simulink library "CarMaker4SL"  (R2021a)
settings: Solver=ode45  StartTime=0.0  StopTime=10.0  RelTol=1e-3
libraries: simulink x1
(part 1 of 3)
settings Model: ModifiedByFormat=IPG  ExtModeAutoUpdateStatusClock=off  Creator=IPG  LastModifiedBy=IPG
settings SolverCC: AlgebraicLoopSolver=TrustRegion
settings DataIOCC: LimitDataPoints=on  SaveFormat=Array  SignalLoggingSaveFormat=ModelDataLogs  ReturnWorkspaceOutputs=off
settings OptimizationCC: BlockReduction=off  BooleanDataType=off  ExpressionDepthLimit=2147483647  LifeSpan=inf
settings DebuggingCC: SaveWithParameterizedLinksMsg=none  UnderspecifiedInitializationDetection=Classic  MergeDetectMultiDrivingBlocksExec=none  SignalResolutionControl=TryResolveAllWithWarning  FcnCallInpInsideContextMsg=warning  StateNameClashWarn=warning  SFUnexpectedBacktrackingDiag=warning  SFNoUnconditionalDefaultTransitionDiag=warning  SFMachineParentedDataDiag=warning  ArithmeticOperatorsInVariantConditions=warning
settings HardwareCC: ProdBitPerPointer=32  ProdBitPerSizeT=32  ProdBitPerPtrDiffT=32  ProdLargestAtomicFloat=None  ProdIntDivRoundTo=Undefined  ProdEndianess=Unspecified  ProdWordSize=32  ProdHWDeviceType=32-bit Generic  TargetUnknown=on
settings ModelReferenceCC: PropagateSignalLabelsOutOfModel=off
settings SFSimCC: SimUseLocalCustomCode=off  CustomCodeUndefinedFunction=UseInterfaceOnly
settings RTWCC: RTWUseLocalCustomCode=off
settings CodeAppCC: StateflowObjectComments=on
settings GRTTargetCC: TargetLangStandard=C89/C90 (ANSI)  CombineOutputUpdateFcns=off  GRTInterface=on
settings ConfigComp: CovMetricSettings=dw  CovSaveCumulativeToWorkspaceVar=on  CovSaveSingleToWorkspaceVar=on  CovExternalEMLEnable=off

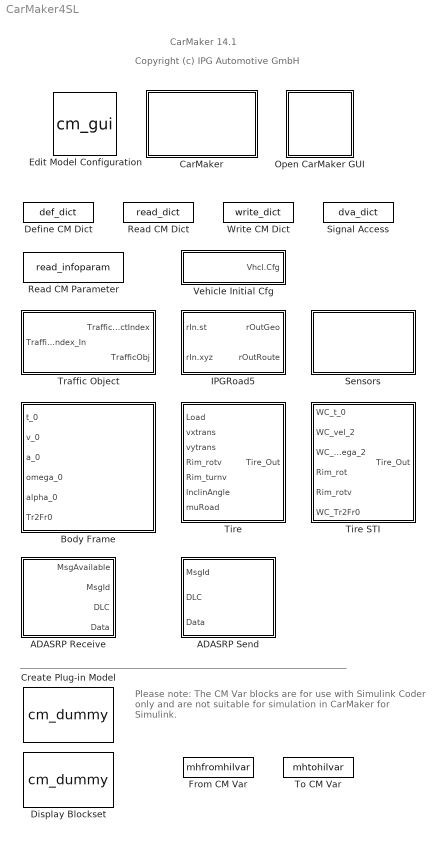
== system CarMaker4SL ==
  note: CarMaker 14.1
  note: Copyright (c) IPG Automotive GmbH
  note: ______________________________________________________________________
  note: Please note:
      | The CM Var blocks are for use with Simulink Coder only
      | and are not suitable for simulation in CarMaker for Simulink.
  ADASRP Receive : Subsystem  mask(ADASRP Receive){xstime=Continuous}
      mask prompts: xstime "Sample time"
      mask help: Receive ADASP CAN message.
      mask TypeOptions xstime: Continuous | Inherited
  ADASRP Send : Subsystem  mask(ADASRP Send){}
      mask help: Send ADASP CAN message.
  Body Frame : Subsystem  mask(Body Frame){xname=[]}
      mask prompts: xname "Body Frame name"
      mask help: Create a body frame on which sensors can be mounted.
      mask Display:
      | fprintf('<< %s >>', xname)
      | port_label('input', 1, 't_0')
      | port_label('input', 2, 'v_0')
      | port_label('input', 3, 'a_0')
      | port_label('input', 4, 'omega_0')
      | port_label('input', 5, 'alpha_0')
      | port_label('input', 6, 'Tr2Fr0')
  CarMaker : Subsystem  TreatAsAtomicUnit=on
      mask Display: image(imread('CarMakerSys.png'));
  Create Plug-in Model : S-Function  FunctionName=cm_dummy  SFunctionDeploymentMode=off  EnableBusSupport=off  mask(Create CarMaker Plug-in Model){}
      settings: OpenFcn=cmPluginModel;
      mask Display: disp('Create\nCarMaker\nPlug-in Model');
  Define CM Dict : S-Function  FunctionName=def_dict  Parameters=xname, xunit, xmono,xtype,xnstates,xfirststate,xinitial,xdvaplace  SFunctionDeploymentMode=off  EnableBusSupport=off  mask(Define CarMaker Dictionary Variable){xname=, xunit=, xmono=off, xtype=Double4, xdvaplace=None, xnstates=0, xfirststate=0, xinitial=0}
      mask prompts: xname "Variable Name"; xunit "Unit"; xmono "Strictly monotone"; xtype "Type"; xdvaplace "DVA write access"; xnstates "Number of states (0=no states)"; xfirststate "First state (if number of states != 0)"; xinitial "Initial value"
      mask help: Define a new variable in the CarMaker data dictionary.
      mask TypeOptions xtype: Double | Double4 | Float | LLong | ULLong | Long | ULong | Int | UInt | Short | UShort | Char | UChar
      mask TypeOptions xdvaplace: None | IO_In | DM | VC | BC | PTC | IO_Out
      mask Display: disp(xname)
  Display Blockset : S-Function  FunctionName=cm_dummy  SFunctionDeploymentMode=off  EnableBusSupport=off
      settings: OpenFcn=open_system('CarMaker4SL')
      mask Display: disp('Display\nCarMaker4SL\nBlockset')
  Edit Model Configuration : S-Function  FunctionName=cm_gui  SFunctionDeploymentMode=off  EnableBusSupport=off
      settings: OpenFcn=cmmodelconf('edit');
      mask Display: image(imread('ModelConfig.png'));
  From CM Var : S-Function  FunctionName=mhfromhilvar  Parameters=xname  SFunctionDeploymentMode=off  EnableBusSupport=off  mask(From CarMaker Var){xname=[]}
      mask prompts: xname "Variable Name"
      mask help:
      | Copy the value of the specified CarMaker C variable to the block's output port.
      |
      | PLEASE NOTE: This block is for use with Simulink Coder only, not for simulation in Simulink.
      mask Display: disp(xname)
  IPGRoad5 : Subsystem  mask(Query IPGRoad){xname=, xevalmode=GeoEval, xconsiderbumps=off, xusepath=off, xwithcurve=off, xabort=on}
      mask prompts: xname "Name"; xevalmode "Mode"; xconsiderbumps "Consider bumps"; xusepath "Use path"; xwithcurve "Output curvature"; xabort "Abort when off road"
      mask help:
      | Query IPGRoad about a given location.
      | The block should be given a unique name. In case of an error this name is logged together with the error message, making it easier to identify the location of the problem.
      mask TypeOptions xevalmode: GeoEval | RouteEval ST | RouteEval XY_S | RouteEval XY_SZ
      mask Display:
      | fprintf('<< %s >>\n%s', xname, xevalmode)
      | port_label('input', 1, 'st')
      | port_label('input', 2, 'xyz')
      | port_label('output', 1, 'Geo')
      | port_label('output', 2, 'Route')
  Open CarMaker GUI : Subsystem  LoadFcn=if ~length(which('cmself')), cmenv; end
      settings: CopyFcn=cmblockmagic('gui_copy')  OpenFcn=cmblockmagic('gui_fix_display'); CM_Simulink
      mask Display: image(imread('CarMakerGUI.png'));
  Read CM Dict : S-Function  FunctionName=read_dict  Parameters=xname, xsync, xstime  SFunctionDeploymentMode=off  EnableBusSupport=off  mask(Read CarMaker Dictionary Variable(s)){xname=, xsync=off, xstime=Continuous}
      mask prompts: xname "Variable Name"; xsync "Show Sync Port"; xstime "Sample time"
      mask help: Copy the value(s) of the specified variable(s) of the CarMaker data dictionary to the block's output port(s). Separate the names of the variables with commas.
      mask TypeOptions xstime: Continuous | Inherited
      mask Display: disp(xname)
  Read CM Parameter : S-Function  FunctionName=read_infoparam  Parameters=xfile,xkey,xnout,xdefaults,[],xmuxed,xstime  SFunctionDeploymentMode=off  EnableBusSupport=off  mask(Read CarMaker Info File Parameter){xfile_type=Vehicle, xfile_instance_vehicle=-, xfile_instance_trailer=1, xfile_instance_general=-, xfile_kind_vehicle=Vehicle, xfile_kind_trailer=Trailer, xfile_kind_general=SimParameters, xfile=Vehicle, xkey=Body.mass, xnout=1, xdefaults=0, xmuxed=on, xstime=Continuous}
      mask prompts: xfile_type "Type"; xfile_instance_vehicle "Instance"; xfile_instance_trailer "Instance"; xfile_instance_general "Instance"; xfile_kind_vehicle "Kind"; xfile_kind_trailer "Kind"; xfile_kind_general "Kind"; xfile "Parameter location"; xkey "Parameter name"; xnout "Number of outputs"; xdefaults "Default value (scalar, vector [...], or empty matrix [ ])"; xmuxed "Muxed output"; xstime "Sample time"
      mask help: Read the first n elements of a CarMaker Info File parameter used in the current Test Run. A default value may be provided in case the parameter does not exist or does not contain at least the specified number of elements. An empty matrix [ ] specified as the default value means the parameter must exist and contain the necessary number of element, otherwise an error is generated.
      mask init:
      | cmupdatemask(gcb, 'ReadCMParameter', 'init');
      mask TypeOptions xfile_type: Vehicle | Trailer | General
      mask Callback xfile_type:
      | cmupdatemask(gcb, 'ReadCMParameter', 'update_TypeOptions');
      |    cmupdatemask(gcb, 'ReadCMParameter', 'set_fileid');
      mask TypeOptions xfile_instance_vehicle: -
      mask Callback xfile_instance_vehicle: cmupdatemask(gcb, 'ReadCMParameter', 'set_fileid');
      mask TypeOptions xfile_instance_trailer: 1 | 2
      mask Callback xfile_instance_trailer: cmupdatemask(gcb, 'ReadCMParameter', 'set_fileid');
      mask TypeOptions xfile_instance_general: -
      mask Callback xfile_instance_general: cmupdatemask(gcb, 'ReadCMParameter', 'set_fileid');
      mask TypeOptions xfile_kind_vehicle: Vehicle | VehicleExtraData | Aero | Brake | BrakeSystem | BrakeControl | Steering | SuspF | SuspR | Susp_FrcSystem | Susp_SpringSystem | Susp_SpringF | Susp_SpringR | Susp_ParasiticStiffnessF | Susp_ParasiticStiffnessR | Susp_ParasiticFrictionF | Susp_ParasiticFrictionR | Susp_TopMountF | Susp_TopMountR | Susp_DamperSystem | Susp_DamperF | Susp_DamperR | Susp_BufferSystem | Susp_BufferF | Susp_BufferR | Susp_StabiSystem | Susp_StabiF | Susp_StabiR | SuspControl | TireFL | TireFR | TireRL | TireRR | PTControl | PTControlOSM | PowerTrain | PowerTrainXWD | PTEngineCU | PTEngine | PTMotorCU | PTMotorISG | PTMotor | PTMotor1 | PTMotor2 | PTMotor3 | PTMotor4 | PTMotor5 | PTMotor6 | PTMotor7 | PTMotor8 | PTMotor9 | PTMotor10 | PTMotor11 | PTTransmCU | PTClutch | PTClutch1 | PTClutch2 | PTClutch3 | PTClutch4 | PTClutch5 | PTClutch6 | PTClutch7 | PTClutch8 | PTClutch9 | PTClutch10 | PTClutch11 | PTGearBox | PTGearBox1 | PTGearBox2 | PTGearBox3 | PTGearBox4 | PTGearBox5 | PTGearBox6 | PTGearBox7 | PTGearBox8 | PTGearBox9 | PTGearBox10 | PTGearBox11 | PTInverter_ISG | PTInverter | PTInverter1 | PTInverter2 | PTInverter3 | PTInverter4 | PTInverter5 | PTInverter6 | PTInverter7 | PTInverter8 | PTInverter9 | PTInverter10 | PTInverter11 | PTDriveLine | PTDriveLineXWD | PTBatteryLV | PTBatteryHV | PTBatteryCU | PTPowerSupply | PTGenCoupling_Front | PTGenCoupling_Rear | PTGenCoupling_Center | PTGenCoupling_Rear2 | PTGenCoupling_Front2 | PTGenCoupling_Rear3 | PTGenCoupling_Rear4 | PTGenCoupling_HangOn | PTGenCoupling_CenterFront | PTGenCoupling_CenterRear | PTUniversalMC | UserDriver | VehicleControl | VhclOperator | SelectorCtrlMapping
      mask Callback xfile_kind_vehicle: cmupdatemask(gcb, 'ReadCMParameter', 'set_fileid');
      mask TypeOptions xfile_kind_trailer: Trailer | Aero | Brake | BrakeSystem | BrakeControl | SuspF | SuspR | SuspM | Susp_FrcSystem | Susp_SpringF | Susp_SpringR | Susp_SpringM | Susp_ParasiticStiffnessF | Susp_ParasiticStiffnessR | Susp_ParasiticStiffnessM | Susp_ParasiticFrictionF | Susp_ParasiticFrictionR | Susp_ParasiticFrictionM | Susp_TopMountF | Susp_TopMountR | Susp_TopMountM | Susp_DamperSystem | Susp_DamperF | Susp_DamperR | Susp_DamperM | Susp_BufferSystem | Susp_BufferF | Susp_BufferR | Susp_BufferM | Susp_StabiSystem | Susp_StabiF | Susp_StabiR | Susp_StabiM | SuspControl | TireFL | TireFR | TireRL | TireRR | TireML | TireMR
      mask Callback xfile_kind_trailer: cmupdatemask(gcb, 'ReadCMParameter', 'set_fileid');
      mask TypeOptions xfile_kind_general: SimParameters | ECUParameters | TestRun | Environment | Road | RadarSensor | Radar_AntGain | CollisionSensor | GNavSensor | TSignSensor | ObjectSensor | LineSensor | RoadSensor | GroundTruthSensor | CameraSensor | ObjByLaneSensor | FSpaceSensor | RSI_MatLib | LidarRSI | LidarRSI_Beams | USonicRSI | USonicRSI_SLobe | RadarRSI | RadarRSI_AntGain | CameraRSI | TestBedParameters
      mask Callback xfile_kind_general: cmupdatemask(gcb, 'ReadCMParameter', 'set_fileid');
      mask TypeOptions xstime: Continuous | Inherited
      mask Display: disp(sprintf('%s\n(%s)', xkey, xfile));
  Sensors : Subsystem
      mask Display: image(imread('SensorSys.png'));
  Signal Access : S-Function  FunctionName=dva_dict  Parameters=xname, xunit, xmono,xtype,xnstates,xfirststate  SFunctionDeploymentMode=off  EnableBusSupport=off  mask(Add CarMaker DVA access to signal.){xname=, xunit=, xmono=off, xtype=Double4, xnstates=0, xfirststate=0}
      mask prompts: xname "Variable Name"; xunit "Unit"; xmono "Strictly monotone"; xtype "Type"; xnstates "Number of states (0=no states)"; xfirststate "First state (if number of states != 0)"
      mask help: The block's input is copied to its output, except when a DVA write access on the given dictionary variable is taking place, in which case the DVA value is copied. The quantity will always contain the signal's current value, so the block also provides a facility for quick signal inspection.
      mask TypeOptions xtype: Double | Double4 | Float | LLong | ULLong | Long | ULong | Int | UInt | Short | UShort | Char | UChar
      mask Display: disp(xname)
  Tire : Subsystem  mask(Tire){xtirepos=FL}
      mask prompts: xtirepos "Tire position"
      mask help:
      | Calculate Contact Point Interface (CPI) tire.
      | This block can only be used in a user defined vehicle.
      mask TypeOptions xtirepos: FL | FR | RL | RR
      mask Display:
      | port_label('input', 1, 'Load')
      | port_label('input', 2, 'vxtrans')
      | port_label('input', 3, 'vytrans')
      | port_label('input', 4, 'Rim_rotv')
      | port_label('input', 5, 'Rim_turnv')
      | port_label('input', 6, 'InclinAngle')
      | port_label('input', 7, 'muRoad')
      | port_label('output', 1, xtirepos)
  Tire STI : Subsystem  mask(Tire){xtirepos=FL}
      mask prompts: xtirepos "Tire position"
      mask help:
      | Calculate Standard Tire Interface (STI) tire.
      | This block can only be used in a user defined vehicle.
      mask TypeOptions xtirepos: FL | FR | RL | RR
      mask Display:
      | port_label('input', 1, 'WC_t_0')
      | port_label('input', 2, 'WC_vel_2')
      | port_label('input', 3, 'WC_omega_2')
      | port_label('input', 4, 'Rim_rot')
      | port_label('input', 5, 'Rim_rotv')
      | port_label('input', 6, 'WC_Tr2Fr0')
      | port_label('output', 1, xtirepos)
  To CM Var : S-Function  FunctionName=mhtohilvar  Parameters=xname  SFunctionDeploymentMode=off  EnableBusSupport=off  mask(To CarMaker Var){xname=[]}
      mask prompts: xname "Variable Name"
      mask help:
      | Copy the value of the block's input port to the specified CarMaker C variable.
      |
      | PLEASE NOTE: This block is for use with Simulink Coder only, not for simulation in Simulink.
      mask Display: disp(xname)
  Traffic Object : Subsystem  mask(CarMaker Traffic Object){xname=INPORT, ximode=Traffic Id, xstime=Continuous}
      mask prompts: xname "Traffic Object (name, index, or INPORT)"; ximode "If used, interpret value from 'toi' inport as"; xstime "Sample time"
      mask help:
      | Read Traffic Object.
      | The traffic object to be read may be specified in one of the following ways: 1. By giving the object's name. 2. By giving the object's numerical index. 3. By using the special name INPORT, so that the object's index is read from the 'toi' inport.
      | The 'TrafficObjectIndex' outport shows either the object's index or -1 if no traffic object with the given name or index exists.
      mask TypeOptions ximode: Traffic Id | Object Id
      mask TypeOptions xstime: Continuous | Inherited
      mask Display:
      | fprintf('<< %s >>', xname)
      | port_label('input', 1, 'toi')
      | port_label('output', 1, 'TrafficObjectIndex')
      | port_label('output', 2, 'TrafficObj')
  Vehicle Initial Cfg : Subsystem  mask(Vehicle Initial Configuration Values){}
      mask help: Provides some initial vehicle configuration values.
  Write CM Dict : S-Function  FunctionName=write_dict  Parameters=xname, xsync, 'off'  SFunctionDeploymentMode=off  EnableBusSupport=off  mask(Write CarMaker Dictionary Variable(s)){xname=, xsync=off}
      mask prompts: xname "Variable Name"; xsync "Show Sync Port"
      mask help: Copy the value(s) of the block's input port to the specified variable(s) of the CarMaker data dictionary. Separate the names of the variables with commas.
      mask Display: disp(xname)

== system CarMaker4SL/ADASRP Receive ==
  ADASRP Recv : S-Function  FunctionName=adasrp_recv  Parameters=xstime  SFunctionDeploymentMode=off  EnableBusSupport=off
  MsgAvailable : Outport  VectorParamsAs1DForOutWhenUnconnected=off
  MsgId : Outport  Port=2  VectorParamsAs1DForOutWhenUnconnected=off
  DLC : Outport  Port=3  VectorParamsAs1DForOutWhenUnconnected=off
  Data : Outport  Port=4  VectorParamsAs1DForOutWhenUnconnected=off
  wires:
  ADASRP Recv/1 -> MsgAvailable/1
  ADASRP Recv/4 -> Data/1
  ADASRP Recv/2 -> MsgId/1
  ADASRP Recv/3 -> DLC/1

== system CarMaker4SL/ADASRP Send ==
  MsgId : Inport
  DLC : Inport  Port=2
  Data : Inport  Port=3
  ADASRP Send : S-Function  FunctionName=adasrp_send  SFunctionDeploymentMode=off  EnableBusSupport=off
  wires:
  MsgId/1 -> ADASRP Send/1
  DLC/1 -> ADASRP Send/2
  Data/1 -> ADASRP Send/3

== system CarMaker4SL/Body Frame ==
  t_0 : Inport
  v_0 : Inport  Port=2
  a_0 : Inport  Port=3
  omega_0 : Inport  Port=4
  alpha_0 : Inport  Port=5
  Tr2Fr0 : Inport  Port=6
  S-Function : S-Function  FunctionName=cm_bdyframe  Parameters=xname  SFunctionDeploymentMode=off  EnableBusSupport=off
  wires:
  t_0/1 -> S-Function/1
  v_0/1 -> S-Function/2
  a_0/1 -> S-Function/3
  omega_0/1 -> S-Function/4
  alpha_0/1 -> S-Function/5
  Tr2Fr0/1 -> S-Function/6

== system CarMaker4SL/CarMaker ==
  CM_FIRST : Subsystem
  CM_LAST : Subsystem
  DrivMan : Subsystem
  Ground : Ground
  IPG Vehicle : Subsystem  TreatAsAtomicUnit=on
  Terminator : Terminator
  VehicleControl : Subsystem
  wires:
  VehicleControl/2(Vhcl.Model.Source) -> IPG Vehicle/2(Vhcl.Model.Source)
  VehicleControl/7(VhclCtrl.PT) -> IPG Vehicle/7(VhclCtrl.PT)
  VehicleControl/6(VhclCtrl.Brake) -> IPG Vehicle/6(VhclCtrl.Brake)
  VehicleControl/5(Vhcl.Misc) -> IPG Vehicle/5(Vhcl.Misc)
  VehicleControl/4(Vhcl.Wheel.In) -> IPG Vehicle/4(Vhcl.Wheel.In)
  VehicleControl/3(VhclCtrl.Steering) -> IPG Vehicle/3(VhclCtrl.Steering)
  VehicleControl/1(Sync_Out) -> IPG Vehicle/1(Sync_In)
  IPG Vehicle/1(Sync_Out) -> CM_LAST/1(Sync_In)
  Ground/1 -> CM_FIRST/1(Sync_In)
  CM_LAST/1(Sync_Out) -> Terminator/1
  CM_FIRST/1(Sync_Out) -> DrivMan/1(Sync_In)
  CM_FIRST/2(Env.Misc) -> DrivMan/2(Env.Misc)
  DrivMan/1(Sync_Out) -> VehicleControl/1(Sync_In)
  DrivMan/2(DrivMan.Out) -> VehicleControl/2(DrivMan.In)

== system CarMaker4SL/IPGRoad5 ==
  rIn.st : Inport
  rIn.xyz : Inport  Port=2
  Bus Creator1 : BusCreator  Inputs=9
  Bus Creator2 : BusCreator  Inputs=22
  Demux1 : Demux  Outputs=9
  Demux3 : Demux  Outputs=22
  S-Function : S-Function  FunctionName=cm_road  Parameters=xname,xevalmode,xconsiderbumps,xusepath,xwithcurve,xabort  SFunctionDeploymentMode=off  EnableBusSupport=off
  rOutGeo : Outport  VectorParamsAs1DForOutWhenUnconnected=off
  rOutRoute : Outport  Port=2  VectorParamsAs1DForOutWhenUnconnected=off
  wires:
  rIn.st/1 -> S-Function/1
  rIn.xyz/1 -> S-Function/2
  Bus Creator2/1 -> rOutRoute/1
  Demux3/1 -> Bus Creator2/1  "x"
  Demux3/2 -> Bus Creator2/2  "y"
  Demux3/3 -> Bus Creator2/3  "z"
  Demux3/4 -> Bus Creator2/4  "nuv x"
  Demux3/5 -> Bus Creator2/5  "nuv y"
  Demux3/6 -> Bus Creator2/6  "nuv z"
  Demux3/7 -> Bus Creator2/7  "suv x"
  Demux3/8 -> Bus Creator2/8  "suv y"
  Demux3/9 -> Bus Creator2/9  "suv z"
  Demux3/10 -> Bus Creator2/10  "tuv x"
  Demux3/11 -> Bus Creator2/11  "tuv y"
  Demux3/12 -> Bus Creator2/12  "tuv z"
  Demux3/14 -> Bus Creator2/14  "t"
  Demux3/13 -> Bus Creator2/13  "s"
  Demux3/15 -> Bus Creator2/15  "curveXY"
  Demux3/16 -> Bus Creator2/16  "width left"
  Demux3/17 -> Bus Creator2/17  "width right"
  Demux3/18 -> Bus Creator2/18  "onRoad"
  Demux3/19 -> Bus Creator2/19  "grade"
  Demux3/20 -> Bus Creator2/20  "slope"
  Demux3/21 -> Bus Creator2/21  "curveZ"
  Demux1/1 -> Bus Creator1/1  "x"
  Demux1/2 -> Bus Creator1/2  "y"
  Demux1/3 -> Bus Creator1/3  "z"
  Demux1/4 -> Bus Creator1/4  "nuv x"
  Demux1/5 -> Bus Creator1/5  "nuv y"
  Demux1/6 -> Bus Creator1/6  "nuv z"
  Demux1/7 -> Bus Creator1/7  "onRoad"
  Demux1/8 -> Bus Creator1/8  "onJunction"
  Demux1/9 -> Bus Creator1/9  "fric"
  Bus Creator1/1 -> rOutGeo/1
  S-Function/1 -> Demux1/1
  S-Function/2 -> Demux3/1
  Demux3/22 -> Bus Creator2/22  "fric"

== system CarMaker4SL/Open CarMaker GUI ==
  S-Function : S-Function  FunctionName=cm_gui  SFunctionDeploymentMode=off  EnableBusSupport=off

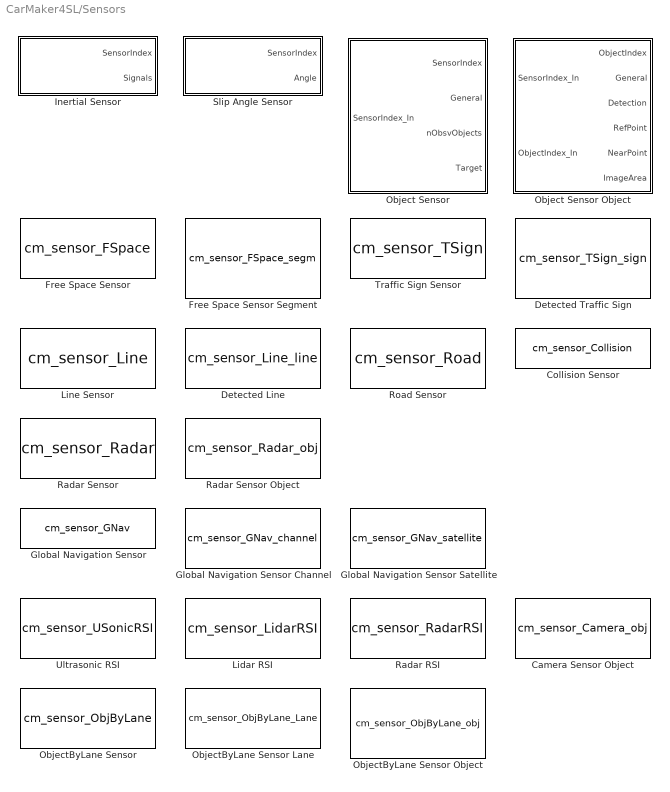
== system CarMaker4SL/Sensors ==
  Camera Sensor Object : S-Function  FunctionName=cm_sensor_Camera_obj  Parameters=xname, xstime  SFunctionDeploymentMode=off  EnableBusSupport=off  mask(Camera Sensor Object){xname=INPORT, xstime=Continuous}
      mask prompts: xname "Camera Sensor (name, index, or INPORT)"; xstime "Sample time"
      mask help:
      | Access sensor specific information about a traffic object.
      | The associated camera sensor may be specified in one of the following ways:
      | 1. By giving the sensor's name.
      | 2. By giving the sensor's numerical index.
      | 3. By using the special name INPORT, so that the sensor's index is read from the 'si' inport.
      | The object index is always read from the 'oi' inport. The 'ObjectIndex' outport shows either the object's index (world object index, see below) or -1 if no camera sensor with the given name or index or no object at the given index exists.
      mask TypeOptions xstime: Continuous | Inherited
      mask Display:
      | fprintf('<< %s >>', xname)
      | port_label('input', 1, 'si')
      | port_label('input', 2, 'oi')
      | port_label('output', 1, 'ObjectIndex')
      | port_label('output', 2, 'Data')
  Collision Sensor : S-Function  FunctionName=cm_sensor_Collision  Parameters=VehicleClass, xstime  SFunctionDeploymentMode=off  EnableBusSupport=off  mask(CarMaker Collision Sensor){VehicleClass=Car, xstime=Continuous}
      mask prompts: xstime "Sample time"
      mask help:
      | Read Collision Sensor data.
      | Returns number of detected collisions and global ID of the collided object for the vehicle body and every wheel.
      mask TypeOptions VehicleClass: Car | MCycle | Truck
      mask TypeOptions xstime: Continuous | Inherited
  Detected Line : S-Function  FunctionName=cm_sensor_Line_line  Parameters=xname, xstime, xside  SFunctionDeploymentMode=off  EnableBusSupport=off  mask(Detected Line){xname=INPORT, xstime=Continuous, xside=left}
      mask prompts: xname "Line Sensor (name, index, or INPORT)"; xstime "Sample time"; xside "Side"
      mask help:
      | Access sensor specific information about a detected line.
      | The associated line sensor may be specified in one of the following ways:
      | 1. By giving the sensor's name.
      | 2. By giving the sensor's numerical index.
      | 3. By using the special name INPORT, so that the sensor's index is read from the 'si' inport.
      | The line index is always read from the 'li' inport. The 'LineIndex' outport shows either the line's index or -1 if no line sensor with the given name or index or no line at the given index exists.
      mask TypeOptions xstime: Continuous | Inherited
      mask TypeOptions xside: left | right
      mask Display:
      | fprintf('<< %s >>', xname)
      | port_label('input', 1, 'si')
      | port_label('input', 2, 'li')
      | port_label('output', 1, 'LineIndex')
      | port_label('output', 2, 'Data')
  Detected Traffic Sign : S-Function  FunctionName=cm_sensor_TSign_sign  Parameters=xname, xstime  SFunctionDeploymentMode=off  EnableBusSupport=off  mask(Detected Traffic Sign){xname=INPORT, xstime=Continuous}
      mask prompts: xname "Traffic Sign Sensor (name, index, or INPORT)"; xstime "Sample time"
      mask help:
      | Access sensor sign information.
      | The associated traffic sign sensor may be specified in one of the following ways:
      | 1. By giving the sensor's name.
      | 2. By giving the sensor's numerical index.
      | 3. By using the special name INPORT, so that the sensor's index is read from the 'si' inport.
      | The sign index is always read from the 'sigi' inport. The 'SignIndex' outport shows either the sign's index or -1 if no traffic sign sensor with the given name or index or no sign at the given index exists.
      mask TypeOptions xstime: Continuous | Inherited
      mask Display:
      | fprintf('<< %s >>', xname)
      | port_label('input', 1, 'si')
      | port_label('input', 2, 'sigi')
      | port_label('output', 1, 'SignIndex')
      | port_label('output', 2, 'Data')
  Free Space Sensor : S-Function  FunctionName=cm_sensor_FSpace  Parameters=xname, xstime  SFunctionDeploymentMode=off  EnableBusSupport=off  mask(Free Space Sensor){xname=INPORT, xstime=Continuous}
      mask prompts: xname "Free Space Sensor (name, index, or INPORT)"; xstime "Sample time"
      mask help:
      | Read Free Space Sensor / Free Space Sensor Plus.
      | The sensor to be read may be specified in one of the following ways:
      | 1. By giving the sensor's name.
      | 2. By giving the sensor's numerical index.
      | 3. By using the special name INPORT, so that the sensor's index is read from the inport.
      | The 'Index' outport shows either the sensor's index or -1 if no free space sensor with the given name or index exists.
      mask TypeOptions xstime: Continuous | Inherited
      mask Display:
      | fprintf('<< %s >>', xname)
      | port_label('input', 1, 'si')
      | port_label('output', 1, 'Index')
      | port_label('output', 2, 'Data')
  Free Space Sensor Segment : S-Function  FunctionName=cm_sensor_FSpace_segm  Parameters=xname, xstime, xplusactive  SFunctionDeploymentMode=off  EnableBusSupport=off  mask(Free Space Sensor Segment){xname=INPORT, xstime=Continuous, xplusactive=off}
      mask prompts: xname "Free Space Sensor (name, index, or INPORT)"; xstime "Sample time"; xplusactive "Free Space Sensor Plus"
      mask help:
      | Access sensor segment information.
      | The associated free space sensor may be specified in one of the following ways:
      | 1. By giving the sensor's name.
      | 2. By giving the sensor's numerical index.
      | 3. By using the special name INPORT, so that the sensor's index is read from the 'si' inport.
      | The segment index is always read from the 'segi' inport. The 'SegmentIndex' outport shows either the segment's index or -1 if no free space sensor with the given name or index or no segment at the given index exists.
      mask TypeOptions xstime: Continuous | Inherited
      mask Display:
      | fprintf('<< %s >>', xname)
      | port_label('input', 1, 'si')
      | port_label('input', 2, 'segi')
      | port_label('output', 1, 'SegmentIndex')
      | port_label('output', 2, 'Data')
  Global Navigation Sensor : S-Function  FunctionName=cm_sensor_GNav  Parameters=xstime  SFunctionDeploymentMode=off  EnableBusSupport=off  mask(Global Navigation Sensor){xstime=Continuous}
      mask prompts: xstime "Sample time"
      mask help:
      | Read Global Navigation Sensor.
      | This block delivers receiver data from the global navigation sensor of CarMaker.
      mask TypeOptions xstime: Continuous | Inherited
  Global Navigation Sensor Channel : S-Function  FunctionName=cm_sensor_GNav_channel  Parameters=channel_idx, xstime  SFunctionDeploymentMode=off  EnableBusSupport=off  mask(Global Navigation Sensor Channel){channel_idx=INPORT, xstime=Continuous}
      mask prompts: channel_idx "Channel (1, 2, ..., 16, or INPORT)"; xstime "Sample time"
      mask help:
      | Access information about a receiver channel.
      | The channel index may be specified in one of the following ways:
      | 1. By giving the channel's numerical index
      | 2. By using the special name INPORT, so that the channel's index is read from the inport.
      mask TypeOptions xstime: Continuous | Inherited
      mask Display:
      | fprintf('<< %s >>', channel_idx)
      | port_label('output', 1, 'Index')
      | port_label('output', 2, 'Data')
      | port_label('input', 1, 'ci')
  Global Navigation Sensor Satellite : S-Function  FunctionName=cm_sensor_GNav_satellite  Parameters=sat_idx, xstime  SFunctionDeploymentMode=off  EnableBusSupport=off  mask(Global Navigation Sensor Satellite){sat_idx=INPORT, xstime=Continuous}
      mask prompts: sat_idx "Satellite (1, 2, ..., 32, or INPORT)"; xstime "Sample time"
      mask help:
      | Access information about a satellite.
      | The satellite index may be specified in one of the following ways:
      | 1. By giving the satellite's numerical index
      | 2. By using the special name INPORT, so that the satellite's index is read from the inport.
      mask TypeOptions xstime: Continuous | Inherited
      mask Display:
      | fprintf('<< %s >>', sat_idx)
      | port_label('output', 1, 'Index')
      | port_label('output', 2, 'Data')
      | port_label('input', 1, 'si')
  Inertial Sensor : Subsystem  mask(Inertial Sensor){xname=[], xstime=Continuous}
      mask prompts: xname "Inertial Sensor (name or index)"; xstime "Sample time"
      mask help:
      | Read Inertial Sensor.
      | The 'SensorIndex' outport shows either the sensor's internal index, or -1 if no inertial sensor with the specified name exists.
      mask TypeOptions xstime: Continuous | Inherited
      mask Display:
      | fprintf('<< %s >>', xname)
      | port_label('output', 1, 'SensorIndex')
      | port_label('output', 2, 'Signals')
  Lidar RSI : S-Function  FunctionName=cm_sensor_LidarRSI  Parameters=xname, xmaxscanpoints, xstime  SFunctionDeploymentMode=off  EnableBusSupport=off  mask(Lidar RSI){xname=INPORT, xmaxscanpoints=10000, xstime=Continuous}
      mask prompts: xname "Lidar RSI (name, index, or INPORT)"; xmaxscanpoints "Maximum number of scan points"; xstime "Sample time"
      mask help:
      | Read Lidar RSI.
      | The sensor to be read may be specified in one of the following ways:
      | 1. By giving the sensor's name.
      | 2. By giving the sensor's numerical index.
      | 3. By using the special name INPORT, so that the sensor's index is read from the inport.
      | The 'Index' outport shows either the sensor's index or -1 if no Lidar RSI with the given name or index exists.
      mask TypeOptions xstime: Continuous | Inherited
      mask Display:
      | fprintf('<< %s >>', xname)
      | port_label('input', 1, 'si')
      | port_label('output', 1, 'Index')
      | port_label('output', 2, 'Data')
  Line Sensor : S-Function  FunctionName=cm_sensor_Line  Parameters=xname, xstime  SFunctionDeploymentMode=off  EnableBusSupport=off  mask(Line Sensor){xname=INPORT, xstime=Continuous}
      mask prompts: xname "Line Sensor (name, index, or INPORT)"; xstime "Sample time"
      mask help:
      | Read Line Sensor.
      | The sensor to be read may be specified in one of the following ways:
      | 1. By giving the sensor's name.
      | 2. By giving the sensor's numerical index.
      | 3. By using the special name INPORT, so that the sensor's index is read from the inport.
      | The 'Index' outport shows either the sensor's index or -1 if no line sensor with the given name or index exists.
      mask TypeOptions xstime: Continuous | Inherited
      mask Display:
      | fprintf('<< %s >>', xname)
      | port_label('input', 1, 'si')
      | port_label('output', 1, 'Index')
      | port_label('output', 2, 'Data')
  Object Sensor : Subsystem  mask(Object Sensor){xname=INPORT, xstime=Continuous}
      mask prompts: xname "Object Sensor (name, index, or INPORT)"; xstime "Sample time"
      mask help:
      | Read Object Sensor.
      | The sensor to be read may be specified in one of the following ways: 1. By giving the sensor's name. 2. By giving the sensor's numerical index. 3. By using the special name INPORT, so that the sensor's index is read from the 'si' inport.
      | The 'SensorIndex' outport shows either the sensor's index or -1 if no object sensor with the given name or index exists.
      mask TypeOptions xstime: Continuous | Inherited
      mask Display:
      | fprintf('<< %s >>', xname)
      | port_label('input', 1, 'si')
      | port_label('output', 1, 'SensorIndex')
      | port_label('output', 2, 'General')
      | port_label('output', 3, 'nObsvObjects')
      | port_label('output', 4, 'Target')
  Object Sensor Object : Subsystem  mask(Object Sensor Object){xname=INPORT, ximode=Observed Objects, xstime=Continuous}
      mask prompts: xname "Object Sensor (name, index, or INPORT)"; ximode "Addressed Objects"; xstime "Sample time"
      mask help:
      | Access sensor specific information about a traffic object.
      | The associated object sensor may be specified in one of the following ways: 1. By giving the sensor's name. 2. By giving the sensor's numerical index. 3. By using the special name INPORT, so that the sensor's index is read from the 'si' inport.
      | The object index is always read from the 'oi' inport. The 'ObjectIndex' outport shows either the object's index (world object index, see below) or -1 if no object sensor with the given name or index or no object at the given index exists.
      | You may use the special object index 99999 to select the sensor's relevant target object.
      | The object index addresses either one of the 'World Objects', i.e. all existing traffic objects, or one of the 'Observed Objects', i.e. the subset of objects inside the sensor's observation radius.
      mask TypeOptions ximode: Observed Objects | World Objects
      mask TypeOptions xstime: Continuous | Inherited
      mask Display:
      | fprintf('<< %s >>', xname)
      | port_label('input', 1, 'si')
      | port_label('input', 2, 'oi')
      | port_label('output', 1, 'ObjectIndex')
      | port_label('output', 2, 'General')
      | port_label('output', 3, 'Detection')
      | port_label('output', 4, 'RefPoint')
      | port_label('output', 5, 'NearPoint')
      | port_label('output', 6, 'ImageArea')
  ObjectByLane Sensor : S-Function  FunctionName=cm_sensor_ObjByLane  Parameters=xname, xstime  SFunctionDeploymentMode=off  EnableBusSupport=off  mask(ObjectByLane Sensor){xname=INPORT, xstime=Continuous}
      mask prompts: xname "ObjectByLane Sensor (name, index, or INPORT)"; xstime "Sample time"
      mask help:
      | Read ObjectByLane Sensor.
      | The sensor to be read may be specified in one of the following ways:
      | 1. By giving the sensor's name.
      | 2. By giving the sensor's numerical index.
      | 3. By using the special name INPORT, so that the sensor's index is read from the inport.
      | The 'Index' outport shows either the sensor's index or -1 if no ObjectByLane sensor with the given name or index exists.
      mask TypeOptions xstime: Continuous | Inherited
      mask Display:
      | fprintf('<< %s >>', xname)
      | port_label('input', 1, 'si')
      | port_label('output', 1, 'Index')
      | port_label('output', 2, 'Data')
  ObjectByLane Sensor Lane : S-Function  FunctionName=cm_sensor_ObjByLane_Lane  Parameters=xname, xstime, xlscope  SFunctionDeploymentMode=off  EnableBusSupport=off  mask(ObjectByLane Sensor Lane){xname=INPORT, xstime=Continuous, xlscope=Left}
      mask prompts: xname "ObjectByLane Sensor Lane (name, index, or INPORT)"; xstime "Sample time"; xlscope "LaneScope"
      mask help:
      | Access sensor specific information about a lane.
      | The associated ObjectByLane sensor may be specified in one of the following ways:
      | 1. By giving the sensor's name.
      | 2. By giving the sensor's numerical index.
      | 3. By using the special name INPORT, so that the sensor's index is read from the 'si' inport.
      | The lane index is always read from the 'li' inport. The 'LaneIndex' outport shows either the lane's index or -1 if no ObjectByLane sensor with the given name or index or no lane at the given index exists.
      mask TypeOptions xstime: Continuous | Inherited
      mask TypeOptions xlscope: Left | Center | Right
      mask Display:
      | fprintf('<< %s >>', xname)
      | port_label('input', 1, 'si')
      | port_label('input', 2, 'li')
      | port_label('output', 1, 'LaneIndex')
      | port_label('output', 2, 'Data')
  ObjectByLane Sensor Object : S-Function  FunctionName=cm_sensor_ObjByLane_obj  Parameters=xname, xstime, xlanescope, xobjlist  SFunctionDeploymentMode=off  EnableBusSupport=off  mask(ObjectByLane Sensor Object){xname=INPORT, xstime=Continuous, xlanescope=Left, xobjlist=Front}
      mask prompts: xname "ObjectByLane Sensor (name, index, or INPORT)"; xstime "Sample time"; xlanescope "Lane Scope"; xobjlist "Object List"
      mask help:
      | Access sensor specific information about a ObjectByLane Sensor object.
      | The associated ObjectByLane sensor may be specified in one of the following ways:
      | 1. By giving the sensor's name.
      | 2. By giving the sensor's numerical index.
      | 3. By using the special name INPORT, so that the sensor's index is read from the 'si' inport.
      | The lane index is always read from the 'li' inport.
      | The object index is always read from the 'oi' inport. The 'ObjectIndex' outport shows either the object's index (world object index, see below) or -1 if no ObjectByLane sensor with the given name or index or no object at the given index exists.
      mask TypeOptions xstime: Continuous | Inherited
      mask TypeOptions xlanescope: Left | Center | Right
      mask TypeOptions xobjlist: Front | Rear
      mask Display:
      | fprintf('<< %s >>', xname)
      | port_label('input', 1, 'si')
      | port_label('input', 2, 'li')
      | port_label('input', 3, 'oi')
      | port_label('output', 1, 'ObjectIndex')
      | port_label('output', 2, 'Data')
  Radar RSI : S-Function  FunctionName=cm_sensor_RadarRSI  Parameters=xname, xmaxdetects, xouttype, xnVRx, xstime  SFunctionDeploymentMode=off  EnableBusSupport=off  mask(Radar RSI){xname=INPORT, xmaxdetects=2000, xouttype=Cartesian, xnVRx=16, xstime=Continuous}
      mask prompts: xname "Radar RSI (name, index, or INPORT)"; xmaxdetects "Maximum number of detections"; xouttype "Output type"; xnVRx "(Maximum) number of virtual receivers"; xstime "Sample time"
      mask help:
      | Read Radar RSI.
      | The sensor to be read may be specified in one of the following ways:
      | 1. By giving the sensor's name.
      | 2. By giving the sensor's numerical index.
      | 3. By using the special name INPORT, so that the sensor's index is read from the inport.
      | The 'Index' outport shows either the sensor's index or -1 if no Radar RSI with the given name or index exists.
      mask Callback xname: cmupdatemask(gcb, 'RadarRSI', 'xname')
      mask TypeOptions xouttype: Cartesian | Spherical | VRx
      mask Callback xouttype: cmupdatemask(gcb, 'RadarRSI', 'xouttype')
      mask TypeOptions xstime: Continuous | Inherited
      mask Display:
      | fprintf('<< %s >>', xname)
      | port_label('input', 1, 'si')
      | port_label('output', 1, 'Index')
      | port_label('output', 2, 'Data')
  Radar Sensor : S-Function  FunctionName=cm_sensor_Radar  Parameters=xname, xstime  SFunctionDeploymentMode=off  EnableBusSupport=off  mask(Radar Sensor){xname=INPORT, xstime=Continuous}
      mask prompts: xname "Radar Sensor (name, index, or INPORT)"; xstime "Sample time"
      mask help:
      | Read Radar Sensor.
      | The sensor to be read may be specified in one of the following ways:
      | 1. By giving the sensor's name.
      | 2. By giving the sensor's numerical index.
      | 3. By using the special name INPORT, so that the sensor's index is read from the inport.
      | The 'Index' outport shows either the sensor's index or -1 if no radar sensor with the given name or index exists.
      mask TypeOptions xstime: Continuous | Inherited
      mask Display:
      | fprintf('<< %s >>', xname)
      | port_label('input', 1, 'si')
      | port_label('output', 1, 'Index')
      | port_label('output', 2, 'Data')
  Radar Sensor Object : S-Function  FunctionName=cm_sensor_Radar_obj  Parameters=xname, ximode, xstime  SFunctionDeploymentMode=off  EnableBusSupport=off  mask(Radar Sensor Object){xname=INPORT, ximode=Observed Objects, xstime=Continuous}
      mask prompts: xname "Radar Sensor (name, index, or INPORT)"; ximode "Addressed Objects"; xstime "Sample time"
      mask help:
      | Access sensor specific information about a traffic object.
      | The associated radar sensor may be specified in one of the following ways:
      | 1. By giving the sensor's name.
      | 2. By giving the sensor's numerical index.
      | 3. By using the special name INPORT, so that the sensor's index is read from the 'si' inport.
      | The object index is always read from the 'oi' inport. The 'ObjectIndex' outport shows either the object's index (world object index, see below) or -1 if no radar sensor with the given name or index or no object at the given index exists.
      | The object index addresses either one of the 'World Objects', i.e. all existing traffic objects, or one of the 'Observed Objects', i.e. the subset of objects inside the sensor's observation radius.
      mask TypeOptions ximode: Observed Objects | World Objects
      mask TypeOptions xstime: Continuous | Inherited
      mask Display:
      | fprintf('<< %s >>', xname)
      | port_label('input', 1, 'si')
      | port_label('input', 2, 'oi')
      | port_label('output', 1, 'ObjectIndex')
      | port_label('output', 2, 'Data')
  Road Sensor : S-Function  FunctionName=cm_sensor_Road  Parameters=xname, xstime  SFunctionDeploymentMode=off  EnableBusSupport=off  mask(Road Sensor){xname=INPORT, xstime=Continuous}
      mask prompts: xname "Road Sensor (name, index, or INPORT)"; xstime "Sample time"
      mask help:
      | Read Road Sensor.
      | The sensor to be read may be specified in one of the following ways:
      | 1. By giving the sensor's name.
      | 2. By giving the sensor's numerical index.
      | 3. By using the special name INPORT, so that the sensor's index is read from the inport.
      | The 'Index' outport shows either the sensor's index or -1 if no road sensor with the given name or index exists.
      mask TypeOptions xstime: Continuous | Inherited
      mask Display:
      | fprintf('<< %s >>', xname)
      | port_label('input', 1, 'si')
      | port_label('output', 1, 'Index')
      | port_label('output', 2, 'Data')
  Slip Angle Sensor : Subsystem  mask(Slip Angle Sensor){xname=[], xstime=Continuous}
      mask prompts: xname "Slip Angle Sensor (name or index)"; xstime "Sample time"
      mask help:
      | Read Slip Angle Sensor.
      | The 'SensorIndex' outport shows either the sensor's internal index, or -1 if no slip angle sensor with the specified name exists.
      mask TypeOptions xstime: Continuous | Inherited
      mask Display:
      | fprintf('<< %s >>', xname)
      | port_label('output', 1, 'SensorIndex')
      | port_label('output', 2, 'Angle')
  Traffic Sign Sensor : S-Function  FunctionName=cm_sensor_TSign  Parameters=xname, xstime  SFunctionDeploymentMode=off  EnableBusSupport=off  mask(Traffic Sign Sensor){xname=INPORT, xstime=Continuous}
      mask prompts: xname "Traffic Sign Sensor (name, index, or INPORT)"; xstime "Sample time"
      mask help:
      | Read Traffic Sign Sensor.
      | The sensor to be read may be specified in one of the following ways:
      | 1. By giving the sensor's name.
      | 2. By giving the sensor's numerical index.
      | 3. By using the special name INPORT, so that the sensor's index is read from the inport.
      | The 'Index' outport shows either the sensor's index or -1 if no traffic sign sensor with the given name or index exists.
      mask TypeOptions xstime: Continuous | Inherited
      mask Display:
      | fprintf('<< %s >>', xname)
      | port_label('input', 1, 'si')
      | port_label('output', 1, 'Index')
      | port_label('output', 2, 'Data')
  Ultrasonic RSI : S-Function  FunctionName=cm_sensor_USonicRSI  Parameters=xname, xmaxreceivers, xmaxdetects, xdistmode, xstime  SFunctionDeploymentMode=off  EnableBusSupport=off  mask(Ultrasonic RSI){xname=INPORT, xmaxreceivers=12, xmaxdetects=1000, xdistmode=Time of Flight, xstime=Continuous}
      mask prompts: xname "Ultrasonic RSI (name, index, or INPORT)"; xmaxreceivers "Maximum number of receivers"; xmaxdetects "Maximum number of detections per receiver"; xdistmode "Distance mode"; xstime "Sample time"
      mask help:
      | Read Ultrasonic RSI.
      | The sensor to be read may be specified in one of the following ways:
      | 1. By giving the sensor's name.
      | 2. By giving the sensor's numerical index.
      | 3. By using the special name INPORT, so that the sensor's index is read from the inport.
      | The 'Index' outport shows either the sensor's index or -1 if no Ultrasonic RSI with the given name or index exists.
      mask TypeOptions xdistmode: Time of Flight | Range
      mask TypeOptions xstime: Continuous | Inherited
      mask Display:
      | fprintf('<< %s >>', xname)
      | port_label('input', 1, 'si')
      | port_label('output', 1, 'Index')
      | port_label('output', 2, 'Data')

== system CarMaker4SL/Tire ==
  Load : Inport
  vxtrans : Inport  Port=2
  vytrans : Inport  Port=3
  Rim_rotv : Inport  Port=4
  Rim_turnv : Inport  Port=5
  InclinAngle : Inport  Port=6
  muRoad : Inport  Port=7
  Bus Creator : BusCreator  Inputs=11
  Demux1 : Demux  Outputs=11
  S-Function : S-Function  FunctionName=cm_tire  Parameters=xtirepos  SFunctionDeploymentMode=off  EnableBusSupport=off
  Tire_Out : Outport  VectorParamsAs1DForOutWhenUnconnected=off
  wires:
  Bus Creator/1 -> Tire_Out/1
  S-Function/1 -> Demux1/1
  Demux1/1 -> Bus Creator/1  "Slp"
  Demux1/2 -> Bus Creator/2  "Alpha"
  Demux1/3 -> Bus Creator/3  "TurnSlp"
  Demux1/4 -> Bus Creator/4  "rBelt_eff"
  Demux1/5 -> Bus Creator/5  "vBelt"
  Demux1/6 -> Bus Creator/6  "LongFrc"
  Demux1/7 -> Bus Creator/7  "SideFrc"
  Demux1/8 -> Bus Creator/8  "LoadFrc"
  Demux1/9 -> Bus Creator/9  "OverturnTrq"
  Demux1/10 -> Bus Creator/10  "RollResist"
  Demux1/11 -> Bus Creator/11  "AlignTrq"
  Load/1 -> S-Function/1
  vxtrans/1 -> S-Function/2
  vytrans/1 -> S-Function/3
  Rim_rotv/1 -> S-Function/4
  Rim_turnv/1 -> S-Function/5
  InclinAngle/1 -> S-Function/6
  muRoad/1 -> S-Function/7

== system CarMaker4SL/Tire STI ==
  WC_t_0 : Inport
  WC_vel_2 : Inport  Port=2
  WC_omega_2 : Inport  Port=3
  Rim_rot : Inport  Port=4
  Rim_rotv : Inport  Port=5
  WC_Tr2Fr0 : Inport  Port=6
  Bus Creator2 : BusCreator  Inputs=26
  Demux1 : Demux  Outputs=26
  S-Function : S-Function  FunctionName=cm_tire_sti  Parameters=xtirepos  SFunctionDeploymentMode=off  EnableBusSupport=off
  Tire_Out : Outport  VectorParamsAs1DForOutWhenUnconnected=off
  wires:
  Bus Creator2/1 -> Tire_Out/1
  S-Function/1 -> Demux1/1
  WC_Tr2Fr0/1 -> S-Function/6
  Rim_rotv/1 -> S-Function/5
  Rim_rot/1 -> S-Function/4
  WC_omega_2/1 -> S-Function/3
  WC_vel_2/1 -> S-Function/2
  WC_t_0/1 -> S-Function/1
  Demux1/26 -> Bus Creator2/26  "P_0 z"
  Demux1/25 -> Bus Creator2/25  "P_0 y"
  Demux1/24 -> Bus Creator2/24  "P_0 x"
  Demux1/23 -> Bus Creator2/23  "muRoad"
  Demux1/22 -> Bus Creator2/22  "Radius"
  Demux1/21 -> Bus Creator2/21  "rBelt_eff"
  Demux1/20 -> Bus Creator2/20  "vBelt"
  Demux1/19 -> Bus Creator2/19  "P_v0_W z"
  Demux1/18 -> Bus Creator2/18  "P_v0_W y"
  Demux1/17 -> Bus Creator2/17  "P_v0_W x"
  Demux1/16 -> Bus Creator2/16  "InclinAngle"
  Demux1/15 -> Bus Creator2/15  "TurnSlp"
  Demux1/14 -> Bus Creator2/14  "Alpha"
  Demux1/13 -> Bus Creator2/13  "Slp"
  Demux1/12 -> Bus Creator2/12  "Trq_W z"
  Demux1/11 -> Bus Creator2/11  "Trq_W y"
  Demux1/10 -> Bus Creator2/10  "Trq_W x"
  Demux1/9 -> Bus Creator2/9  "Frc_W z"
  Demux1/8 -> Bus Creator2/8  "Frc_W y"
  Demux1/7 -> Bus Creator2/7  "Frc_W x"
  Demux1/6 -> Bus Creator2/6  "Trq_C z"
  Demux1/5 -> Bus Creator2/5  "Trq_C y"
  Demux1/4 -> Bus Creator2/4  "Trq_C x"
  Demux1/3 -> Bus Creator2/3  "Frc_C z"
  Demux1/2 -> Bus Creator2/2  "Frc_C y"
  Demux1/1 -> Bus Creator2/1  "Frc_C x"

== system CarMaker4SL/Traffic Object ==
  TrafficObjectIndex_In : Inport
  Bus Creator : BusCreator  Inputs=30
  Demux : Demux  Outputs=30
      settings: DisplayOption=none
  S-Function : S-Function  FunctionName=cm_obstacle  Parameters=xname, ximode, xstime  SFunctionDeploymentMode=off  EnableBusSupport=off
  TrafficObjectIndex : Outport  VectorParamsAs1DForOutWhenUnconnected=off
  TrafficObj : Outport  Port=2  VectorParamsAs1DForOutWhenUnconnected=off
  wires:
  Demux/28 -> Bus Creator/28  "a_0 z"
  Demux/27 -> Bus Creator/27  "a_0 y"
  Demux/26 -> Bus Creator/26  "a_0 x"
  Demux/25 -> Bus Creator/25  "v_0 z"
  Demux/24 -> Bus Creator/24  "v_0 y"
  Demux/23 -> Bus Creator/23  "v_0 x"
  Demux/22 -> Bus Creator/22  "Tr2Fr0 2 2"
  Demux/21 -> Bus Creator/21  "Tr2Fr0 2 1"
  Demux/20 -> Bus Creator/20  "Tr2Fr0 2 0"
  Demux/19 -> Bus Creator/19  "Tr2Fr0 1 2"
  Demux/18 -> Bus Creator/18  "Tr2Fr0 1 1"
  Demux/17 -> Bus Creator/17  "Tr2Fr0 1 0"
  Demux/16 -> Bus Creator/16  "Tr2Fr0 0 2"
  Demux/15 -> Bus Creator/15  "Tr2Fr0 0 1"
  Demux/14 -> Bus Creator/14  "Tr2Fr0 0 0"
  Demux/13 -> Bus Creator/13  "r_zyx z"
  Demux/12 -> Bus Creator/12  "r_zyx y"
  Demux/11 -> Bus Creator/11  "r_zyx x"
  Demux/10 -> Bus Creator/10  "t_0 z"
  Demux/9 -> Bus Creator/9  "t_0 y"
  Demux/8 -> Bus Creator/8  "t_0 x"
  Demux/7 -> Bus Creator/7  "LatVel"
  Demux/6 -> Bus Creator/6  "LongAcc"
  Demux/5 -> Bus Creator/5  "LongVel"
  Demux/4 -> Bus Creator/4  "tRoad"
  Demux/3 -> Bus Creator/3  "sRoad"
  Demux/2 -> Bus Creator/2  "DetectLevel"
  Demux/1 -> Bus Creator/1  "State"
  TrafficObjectIndex_In/1 -> S-Function/1
  S-Function/1 -> TrafficObjectIndex/1
  Bus Creator/1 -> TrafficObj/1
  S-Function/2 -> Demux/1
  Demux/29 -> Bus Creator/29  "TrafficObjectId"
  Demux/30 -> Bus Creator/30  "GlobalObjectId"

== system CarMaker4SL/Vehicle Initial Cfg ==
  CreateBus Vhcl.Cfg : Subsystem
  VehicleControlUpd : S-Function  FunctionName=cm_initial  SFunctionDeploymentMode=off  EnableBusSupport=off
  Vhcl.Cfg : Outport  VectorParamsAs1DForOutWhenUnconnected=off
  wires:
  CreateBus Vhcl.Cfg/1(Out1) -> Vhcl.Cfg/1
  VehicleControlUpd/1 -> CreateBus Vhcl.Cfg/1(In1)
